simulink model "DPSK_7"  (R2018a)
settings: Solver=VariableStepAuto  StartTime=0.0  StopTime=10000  RelTol=1e-3
values from neighbouring files (symbols this model uses):
  SymbolRate = 2    [DPSK_77.m]    (also in FSK_11.m = 1000; PAM_22.m; PSK_44.m)
libraries: commutil2 x4, commsink2 x2, commchan3 x1, commdigbbndpm3 x1, commrandsrc3 x1, commdigbbndam3 x1
settings Model: Creator=sdf  LastModifiedBy=sdf

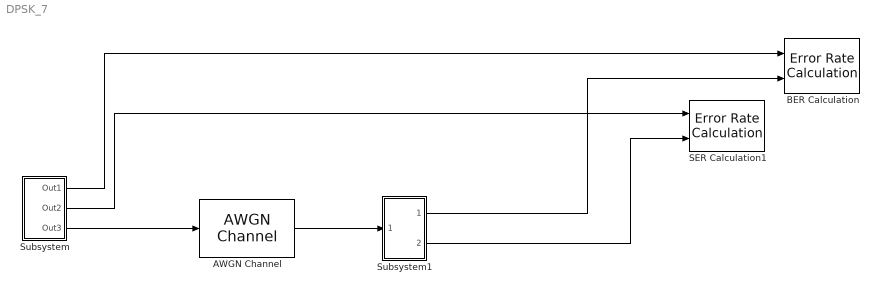
== system DPSK_7 ==
  AWGN Channel : commchan3/AWGN Channel  InputProcessing=Columns as channels (frame based)  seed=1111  noiseMode="Signal to noise ratio  (Es/No)"  EbNodB=10  EsNodB=SNR  SNRdB=10  bitsPerSym=1  Ps=1  Tsym=1/SymbolRate  variance=1
  BER Calculation : commsink2/Error Rate Calculation  N=0  st_delay=2*SymbolRate  cp_mode=Entire frame  subframe=[]  PMode=Workspace  WsName=BER  RsMode2=off  stop=off  numErr=100  maxBits=1e6
  SER Calculation1 : commsink2/Error Rate Calculation  N=0  st_delay=SymbolRate  cp_mode=Entire frame  subframe=[]  PMode=Workspace  WsName=SER  RsMode2=off  stop=off  numErr=100  maxBits=1e6
  Subsystem : Subsystem
  Subsystem1 : Subsystem
  wires:
  Subsystem/1(Out1) -> BER Calculation/1
  Subsystem/2(Out2) -> SER Calculation1/1
  Subsystem/3(Out3) -> AWGN Channel/1
  AWGN Channel/1 -> Subsystem1/1(In1)
  Subsystem1/1(Out1) -> BER Calculation/2
  Subsystem1/2(Out2) -> SER Calculation1/2

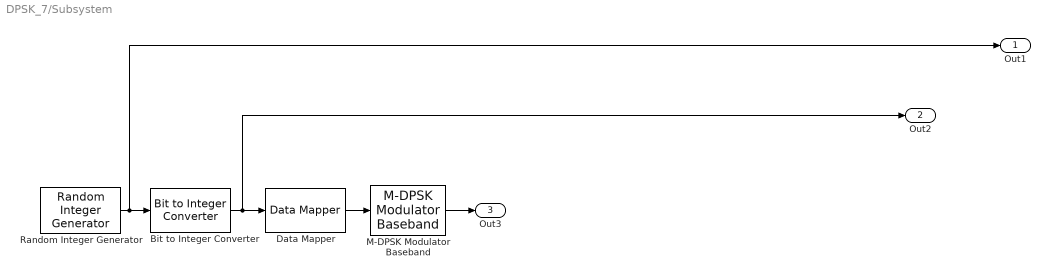
== system DPSK_7/Subsystem ==
  Bit to Integer Converter : commutil2/Bit to Integer Converter  nbits=2  bitOrder=MSB first  signedOutputValues=Unsigned  outDtype=Inherit via internal rule  outDtypeSigned=Inherit via internal rule
  Data Mapper : commutil2/Data Mapper  MapMode=Binary to Gray  M=4  MapVec=[0 1 3 2 7 6 4 5]
      settings: SourceProductName=Communications System Toolbox  SourceProductBaseCode=CM
  M-DPSK Modulator Baseband : commdigbbndpm3/M-DPSK Modulator Baseband  M=4  InType=Integer  Enc=Binary  Ph=0  outDtype=double
      settings: SourceProductName=Communications System Toolbox  SourceProductBaseCode=CM
  Random Integer Generator : commrandsrc3/Random Integer Generator  SetSize=2  SeedSource=Parameter  Seed=37  SampleTime=1/(2*SymbolRate)  SamplesPerFrame=2*SymbolRate  OutputDataType=double  SimulateUsing=Interpreted execution
  Out1 : Outport
  Out2 : Outport  Port=2
  Out3 : Outport  Port=3
  wires:
  Data Mapper/1 -> M-DPSK Modulator Baseband/1
  Bit to Integer Converter/1 -> Out2/1, Data Mapper/1
  Random Integer Generator/1 -> Out1/1, Bit to Integer Converter/1
  M-DPSK Modulator Baseband/1 -> Out3/1

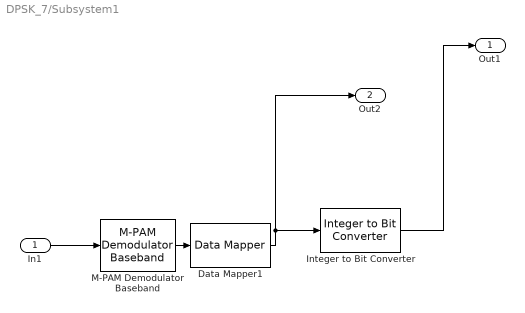
== system DPSK_7/Subsystem1 ==
  In1 : Inport
  Data Mapper1 : commutil2/Data Mapper  MapMode=Binary to Gray  M=4  MapVec=[0 1 3 2 7 6 4 5]
      settings: SourceProductName=Communications System Toolbox  SourceProductBaseCode=CM
  Integer to Bit Converter : commutil2/Integer to Bit Converter  nbits=2  signedInputValues=Unsigned  bitOrder=MSB first  outDtype=Inherit via internal rule
  M-PAM Demodulator Baseband : commdigbbndam3/M-PAM Demodulator Baseband  M=4  OutType=Integer  Dec=Binary  PowType=Min. distance between symbols  MinDist=2  AvgPow=1  PeakPow=1  outDtype1=Inherit via internal rule  outDtype2=Inherit via internal rule  denormFactorWordLen=16  denormFactorDataTypeStr=Inherit: Same word length as input  denormFactorLastDataTypeStr=Inherit: Same word length as input  prodOutWordLen=16  prodOutRoundingMode=Floor  prodOutOverflowMode=Wrap  prodOutOvFlMode=off  prodOutOvFlModeLastStrValue=off  sumWordLen=16
      settings: SourceProductName=Communications System Toolbox  SourceProductBaseCode=CM
  Out1 : Outport
  Out2 : Outport  Port=2
  wires:
  Integer to Bit Converter/1 -> Out1/1
  M-PAM Demodulator Baseband/1 -> Data Mapper1/1
  Data Mapper1/1 -> Out2/1, Integer to Bit Converter/1
  In1/1 -> M-PAM Demodulator Baseband/1
